simulink model "Version_finale"  (R2025b)
settings: Solver=VariableStepAuto  StartTime=0.0  StopTime=10.0  RelTol=1e-3
undefined symbols (not defined in the file): dspblkCoreblockFVToolHelper, gcbh
settings Model: Creator=elio  LastModifiedBy=elio

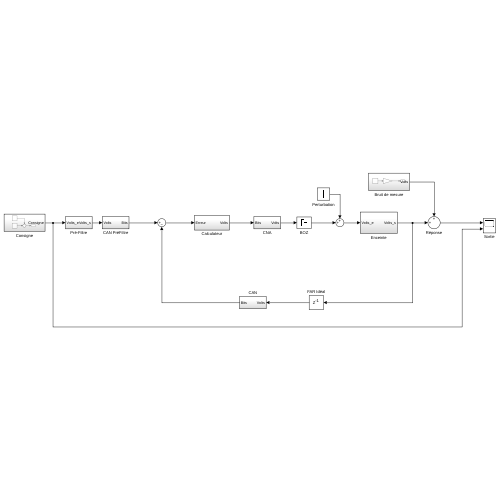
[thumbnail: Simulink's stored preview of the top-level diagram]
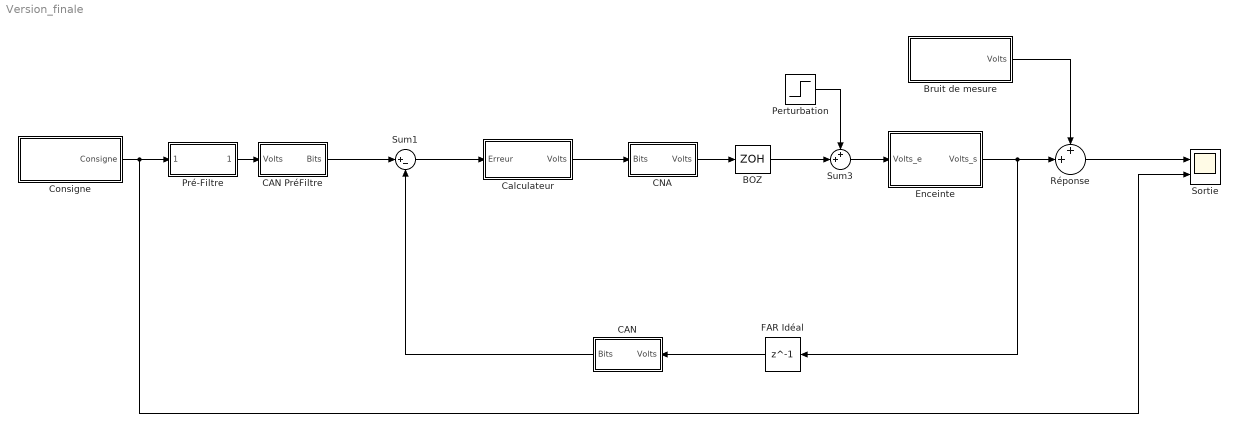
== system Version_finale ==
  BOZ : ZeroOrderHold  SampleTime=0.01
  Bruit de mesure : Subsystem
  CAN : Subsystem
  CAN PréFiltre : Subsystem
  CNA : Subsystem
  Calculateur : Subsystem
  Consigne : Subsystem
  Enceinte : Subsystem
  FAR Idéal : Delay  DelayLength=1  InitialCondition=0  SampleTime=0.01
  Perturbation : Step  Time=2  SampleTime=0.01
  Pré-Filtre : Subsystem
  Réponse : Sum  Inputs=++|
  Sortie : Scope  NumInputPorts=2
      settings: ActiveDisplayYMinimum=0.76584614760366221  ActiveDisplayYMaximum=2.9120450440842305
  Sum1 : Sum  Inputs=|+-
  Sum3 : Sum  Inputs=++|
  wires:
  Enceinte/1(Volts_s) -> Réponse/2, FAR Idéal/1
  Réponse/1 -> Sortie/1
  CNA/1(Volts) -> BOZ/1
  Calculateur/1(Volts) -> CNA/1(Bits)
  BOZ/1 -> Sum3/2
  Sum3/1 -> Enceinte/1(Volts_e)
  Sum1/1 -> Calculateur/1(Erreur)
  Pré-Filtre/1(Volts_s) -> CAN PréFiltre/1(Volts)
  Consigne/1(Consigne) -> Sortie/2, Pré-Filtre/1(Volts_e)
  CAN/1(Bits) -> Sum1/2
  FAR Idéal/1 -> CAN/1(Volts)
  CAN PréFiltre/1(Bits) -> Sum1/1
  Perturbation/1 -> Sum3/1
  Bruit de mesure/1(Volts) -> Réponse/1

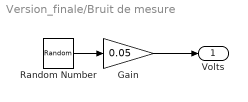
== system Version_finale/Bruit de mesure ==
  Gain : Gain  Gain=0.05
  Random Number : RandomNumber  Variance=0.5  SampleTime=0.01
  Volts : Outport
  wires:
  Random Number/1 -> Gain/1
  Gain/1 -> Volts/1

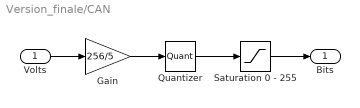
== system Version_finale/CAN ==
  Volts : Inport
  Gain : Gain  Gain=256/5  SaturateOnIntegerOverflow=on  OutDataTypeStr=Inherit: Same as input  ParamDataTypeStr=Inherit: Same as input
  Quantizer : Quantizer  QuantizationInterval=1
  Saturation 0 - 255 : Saturate  UpperLimit=255  LowerLimit=0
  Bits : Outport
  wires:
  Gain/1 -> Quantizer/1
  Volts/1 -> Gain/1
  Quantizer/1 -> Saturation 0 - 255/1
  Saturation 0 - 255/1 -> Bits/1

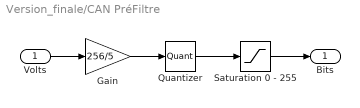
== system Version_finale/CAN PréFiltre ==
  Volts : Inport
  Gain : Gain  Gain=256/5  SaturateOnIntegerOverflow=on  OutDataTypeStr=Inherit: Same as input  ParamDataTypeStr=Inherit: Same as input
  Quantizer : Quantizer  QuantizationInterval=1
  Saturation 0 - 255 : Saturate  UpperLimit=255  LowerLimit=0
  Bits : Outport
  wires:
  Gain/1 -> Quantizer/1
  Volts/1 -> Gain/1
  Quantizer/1 -> Saturation 0 - 255/1
  Saturation 0 - 255/1 -> Bits/1

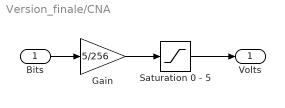
== system Version_finale/CNA ==
  Bits : Inport
  Gain : Gain  Gain=5/256  SaturateOnIntegerOverflow=on  OutDataTypeStr=Inherit: Same as input  ParamDataTypeStr=Inherit: Same as input
  Saturation 0 - 5 : Saturate  UpperLimit=5  LowerLimit=0
  Volts : Outport
  wires:
  Bits/1 -> Gain/1
  Gain/1 -> Saturation 0 - 5/1
  Saturation 0 - 5/1 -> Volts/1

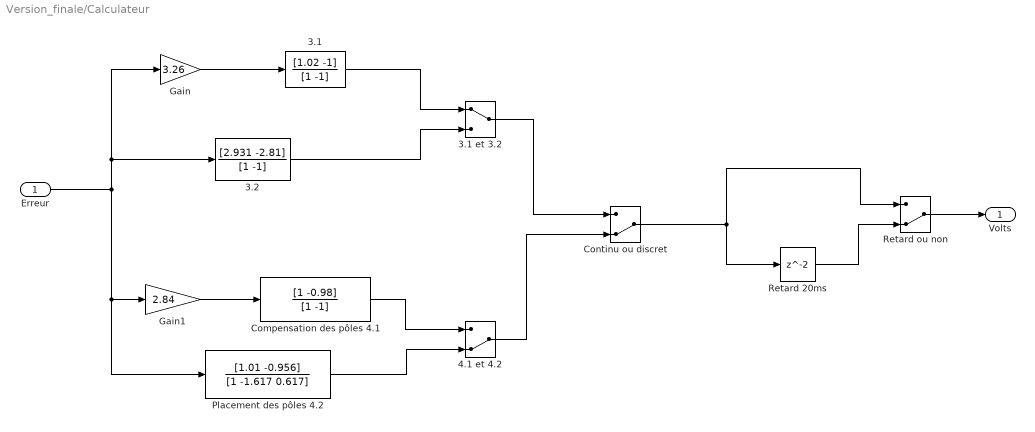
== system Version_finale/Calculateur ==
  Erreur : Inport
  3.1 : DiscreteFilter  LoadFcn=dspblkCoreblockFVToolHelper(gcbh,'load');  Numerator=[1.02 -1]  Denominator=[1 -1]  SampleTime=0.01
      settings: CopyFcn=dspblkCoreblockFVToolHelper(gcbh,'copy');  DeleteFcn=dspblkCoreblockFVToolHelper(gcbh,'close');  ModelCloseFcn=dspblkCoreblockFVToolHelper(gcbh,'close');  PreSaveFcn=dspblkCoreblockFVToolHelper(gcbh,'presave');  PostSaveFcn=dspblkCoreblockFVToolHelper(gcbh,'postsave');  CloseFcn=dspblkCoreblockFVToolHelper(gcbh,'close');
  3.1 et 3.2 : ManualSwitch
  3.2 : DiscreteFilter  LoadFcn=dspblkCoreblockFVToolHelper(gcbh,'load');  Numerator=[2.931 -2.81]  Denominator=[1 -1]  SampleTime=0.01
      settings: CopyFcn=dspblkCoreblockFVToolHelper(gcbh,'copy');  DeleteFcn=dspblkCoreblockFVToolHelper(gcbh,'close');  ModelCloseFcn=dspblkCoreblockFVToolHelper(gcbh,'close');  PreSaveFcn=dspblkCoreblockFVToolHelper(gcbh,'presave');  PostSaveFcn=dspblkCoreblockFVToolHelper(gcbh,'postsave');  CloseFcn=dspblkCoreblockFVToolHelper(gcbh,'close');
  4.1 et 4.2 : ManualSwitch  CurrentSetting=0
  Compensation des pôles 4.1 : DiscreteFilter  LoadFcn=dspblkCoreblockFVToolHelper(gcbh,'load');  Numerator=[1 -0.98]  Denominator=[1 -1]  SampleTime=0.01
      settings: CopyFcn=dspblkCoreblockFVToolHelper(gcbh,'copy');  DeleteFcn=dspblkCoreblockFVToolHelper(gcbh,'close');  ModelCloseFcn=dspblkCoreblockFVToolHelper(gcbh,'close');  PreSaveFcn=dspblkCoreblockFVToolHelper(gcbh,'presave');  PostSaveFcn=dspblkCoreblockFVToolHelper(gcbh,'postsave');  CloseFcn=dspblkCoreblockFVToolHelper(gcbh,'close');
  Continu ou discret : ManualSwitch  CurrentSetting=0
  Gain : Gain  Gain=3.26
  Gain1 : Gain  Gain=2.84
  Placement des pôles 4.2 : DiscreteFilter  LoadFcn=dspblkCoreblockFVToolHelper(gcbh,'load');  Numerator=[1.01 -0.956]  Denominator=[1 -1.617 0.617]  SampleTime=0.01
      settings: CopyFcn=dspblkCoreblockFVToolHelper(gcbh,'copy');  DeleteFcn=dspblkCoreblockFVToolHelper(gcbh,'close');  ModelCloseFcn=dspblkCoreblockFVToolHelper(gcbh,'close');  PreSaveFcn=dspblkCoreblockFVToolHelper(gcbh,'presave');  PostSaveFcn=dspblkCoreblockFVToolHelper(gcbh,'postsave');  CloseFcn=dspblkCoreblockFVToolHelper(gcbh,'close');
  Retard 20ms : Delay  InitialCondition=0  SampleTime=0.01
  Retard ou non : ManualSwitch  CurrentSetting=0
  Volts : Outport
  wires:
  Erreur/1 -> 3.2/1, Gain/1, Gain1/1, Placement des pôles 4.2/1
  Gain/1 -> 3.1/1
  3.1 et 3.2/1 -> Continu ou discret/1
  Placement des pôles 4.2/1 -> 4.1 et 4.2/2
  4.1 et 4.2/1 -> Continu ou discret/2
  Continu ou discret/1 -> Retard ou non/1, Retard 20ms/1
  Retard ou non/1 -> Volts/1
  Retard 20ms/1 -> Retard ou non/2
  3.1/1 -> 3.1 et 3.2/1
  3.2/1 -> 3.1 et 3.2/2
  Gain1/1 -> Compensation des pôles 4.1/1
  Compensation des pôles 4.1/1 -> 4.1 et 4.2/1

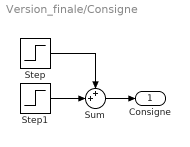
== system Version_finale/Consigne ==
  Step : Step  Time=4  After=-0.5  SampleTime=0.01
  Step1 : Step  Time=0.5  Before=1.66  After=2.33  SampleTime=0.01
  Sum : Sum  Inputs=++|
  Consigne : Outport
  wires:
  Step/1 -> Sum/1
  Step1/1 -> Sum/2
  Sum/1 -> Consigne/1

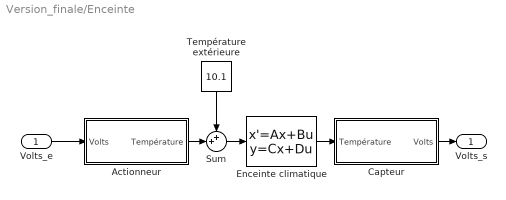
== system Version_finale/Enceinte ==
  Volts_e : Inport
  Actionneur : Subsystem
  Capteur : Subsystem
  Enceinte climatique : StateSpace  A=-2  B=2  D=0  InitialCondition=9.95
  Sum : Sum  Inputs=++|
  Température extérieure : Constant  Value=10.1
  Volts_s : Outport
  wires:
  Volts_e/1 -> Actionneur/1(Volts)
  Sum/1 -> Enceinte climatique/1
  Actionneur/1(Température) -> Sum/2
  Température extérieure/1 -> Sum/1
  Enceinte climatique/1 -> Capteur/1(Température)
  Capteur/1(Volts) -> Volts_s/1

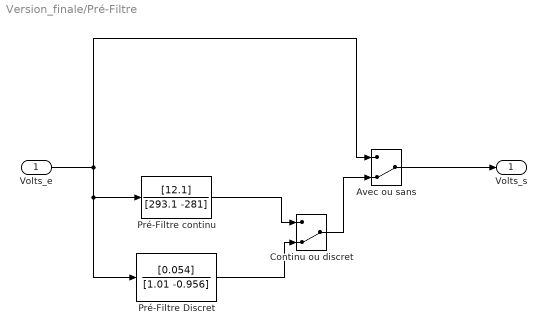
== system Version_finale/Pré-Filtre ==
  Volts_e : Inport
  Avec ou sans : ManualSwitch  CurrentSetting=0
  Continu ou discret : ManualSwitch  CurrentSetting=0
  Pré-Filtre Discret : DiscreteFilter  LoadFcn=dspblkCoreblockFVToolHelper(gcbh,'load');  Numerator=[0.054]  Denominator=[1.01 -0.956]  SampleTime=0.01
      settings: CopyFcn=dspblkCoreblockFVToolHelper(gcbh,'copy');  DeleteFcn=dspblkCoreblockFVToolHelper(gcbh,'close');  ModelCloseFcn=dspblkCoreblockFVToolHelper(gcbh,'close');  PreSaveFcn=dspblkCoreblockFVToolHelper(gcbh,'presave');  PostSaveFcn=dspblkCoreblockFVToolHelper(gcbh,'postsave');  CloseFcn=dspblkCoreblockFVToolHelper(gcbh,'close');
  Pré-Filtre continu : DiscreteFilter  LoadFcn=dspblkCoreblockFVToolHelper(gcbh,'load');  Numerator=[12.1]  Denominator=[293.1 -281]  SampleTime=0.01
      settings: CopyFcn=dspblkCoreblockFVToolHelper(gcbh,'copy');  DeleteFcn=dspblkCoreblockFVToolHelper(gcbh,'close');  ModelCloseFcn=dspblkCoreblockFVToolHelper(gcbh,'close');  PreSaveFcn=dspblkCoreblockFVToolHelper(gcbh,'presave');  PostSaveFcn=dspblkCoreblockFVToolHelper(gcbh,'postsave');  CloseFcn=dspblkCoreblockFVToolHelper(gcbh,'close');
  Volts_s : Outport
  wires:
  Volts_e/1 -> Pré-Filtre Discret/1, Pré-Filtre continu/1, Avec ou sans/1
  Avec ou sans/1 -> Volts_s/1
  Pré-Filtre continu/1 -> Continu ou discret/1
  Continu ou discret/1 -> Avec ou sans/2
  Pré-Filtre Discret/1 -> Continu ou discret/2

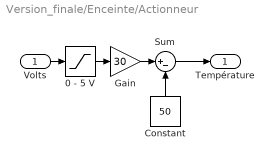
== system Version_finale/Enceinte/Actionneur ==
  Volts : Inport
  "0 - 5 V " : Saturate  UpperLimit=5  LowerLimit=0
  Constant : Constant  Value=50
  Gain : Gain  Gain=30
  Sum : Sum  Inputs=|+-
  Température : Outport
  wires:
  Volts/1 -> "0 - 5 V "/1
  "0 - 5 V "/1 -> Gain/1
  Gain/1 -> Sum/1
  Constant/1 -> Sum/2
  Sum/1 -> Température/1

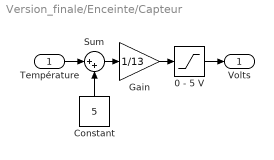
== system Version_finale/Enceinte/Capteur ==
  Température : Inport
  "0 - 5 V " : Saturate  UpperLimit=5  LowerLimit=0
  Constant : Constant  Value=5
  Gain : Gain  Gain=1/13
  Sum : Sum  Inputs=|++
  Volts : Outport
  wires:
  Constant/1 -> Sum/2
  Température/1 -> Sum/1
  Sum/1 -> Gain/1
  Gain/1 -> "0 - 5 V "/1
  "0 - 5 V "/1 -> Volts/1
